simulink model "sampleModel1763"  (R2023a)
settings: Solver=VariableStepAuto  StartTime=0.0  StopTime=10.0  RelTol=1e-3
libraries: hdlsllib x4, simulink x1
settings Model: Creator=user1  LastModifiedBy=user1

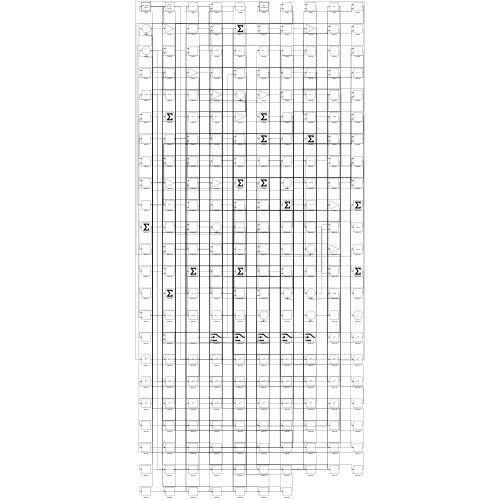
[thumbnail: Simulink's stored preview of the top-level diagram]
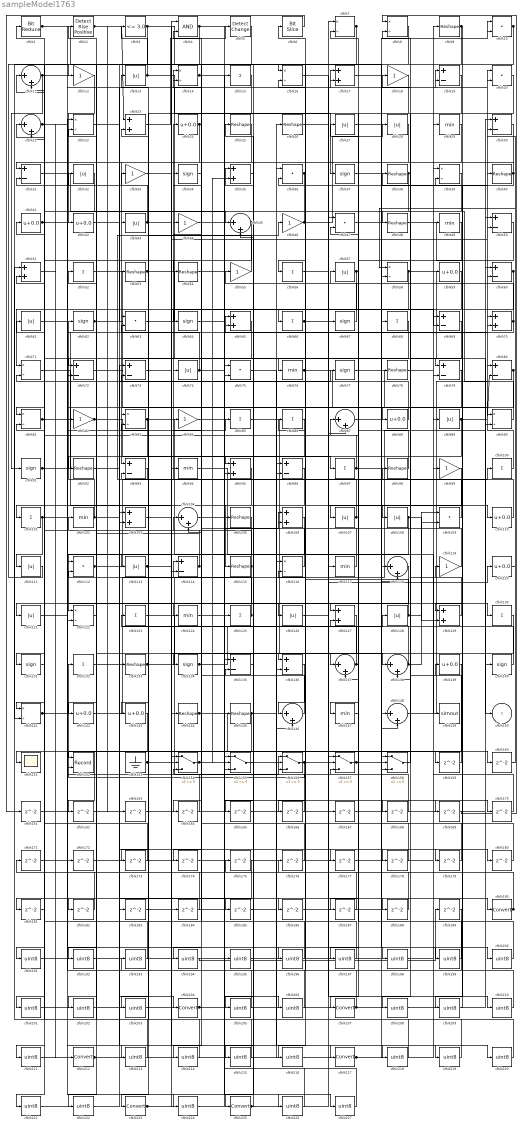
== system sampleModel1763 ==
  cfblk1 : hdlsllib/Logic and Bit Operations/Bit Reduce  mode=AND
  cfblk{10,20,36,47,63,75,109,112} (8 alike) : DotProduct  OutDataTypeStr=Inherit: Inherit via internal rule
  cfblk{15,52,56,66,68,85..86,97,100..101,123,125,130,132} (14 alike) : Sum  Inputs=+
  cfblk{29,49,76,94,102,117,124,147} (8 alike) : MinMax
  cfblk{17,23,35,51,65,70,95,103,106,127,129,136} (12 alike) : Sum
  cfblk{11,21,45,87,104,118,137..138,146,148} (10 alike) : Sum  Inputs=|++
  cfblk{9,25..26,38,40,48,53..54,78,92,98,105,115,133,144..145} (16 alike) : Reshape
  cfblk{13,27..28,32,43,57,61,74,89,107..108,111,113,121,126,128} (16 alike) : Abs  SaturateOnIntegerOverflow=off
  cfblk{24,41..42,59,88,110,120,139,142..143} (10 alike) : Bias  Bias=0.0  SaturateOnIntegerOverflow=off
  cfblk{19,30..31,50,60,69,72..73,79..80,93,96,114,135} (14 alike) : Sum  Inputs=+-
  cfblk{7..8,14,16,22,39,58,71,81,83,90,116,122,141} (14 alike) : Product  Inputs=*/  RndMeth=Zero  SaturateOnIntegerOverflow=on
  cfblk{12,18,33,44,46,55,82,84,99,119} (10 alike) : Gain
  cfblk{34,37,62,64,67,77,91,131,134,140} (10 alike) : Signum
  cfblk149 : ToWorkspace  VariableName=simout  SaveFormat=Timeseries  SampleTime=-1
  cfblk151 : Scope
  cfblk152 : Record  FileSettingsInternal="{\"entries\":[{\"content\":{\"excelSettings\":{\"content\":{},\"type\":\"Streamout.ExcelSettings\"}},\"type\":\"Streamout.FileSettingStorage\",\"uuid\":\"\"}],\"packageUris\":[\"http:\\/\\/schema.mathworks.com\\/mf0\\/streamout_blocks\\/R2020a\"],\"version\":\"1.0\"}"  Layout=[1 1]  SignalsInternal="{\"entries\":[{\"content\":{\"signals\":[{\"content\":{\"blockPath\":[],\"dimensions\":[1],\"domain\":\"\",\"lineColor\":\"#a2142f\",\"plots\":[1],\"port\":1,\"signalID\":3829,\"signalName\":\"XY Graph:1\"},\"type\":\"RecordBlkView.Signal\",\"uuid\":\"\"},{\"content\":{\"blockPath\":[],\"dimensions\":[1],\"domain\":\"\",\"lineColor\":\"#139fff\",\"plots\":[1],\"port\":2,\"signalID\":3832,\"signalName\":\"XY Graph:2\"},\"type\":\"RecordBlkView.Signal\",\"uuid\":\"\"}]},\"type\":\"RecordBlkView.InputSignals\",\"uuid\":\"\"}],\"packageUris\":[\"http:\\/\\/schema.mathworks.com\\/mf0\\/streamout_blocks\\/R2020a\"],\"version\":\"1.0\"}"  VisualizationBindings="{\"xyplotplugin\":{\"info\":[{\"series\":[{\"bindingParametersList\":[{\"parameter\":\"X-Axis\",\"signalID\":3829,\"signalName\":\"XY Graph:1\"},{\"parameter\":\"Y-Axis\",\"signalID\":3832,\"signalName\":\"XY Graph:2\"}],\"seriesID\":32770}],\"subplotID\":1}]}}"  CompatibilityTag=XY  st=-1
  cfblk153 : Ground
  cfblk{154..158} (5 alike) : Switch  SaturateOnIntegerOverflow=off  InputSameDT=off
  cfblk{159..189} (31 alike) : Delay  SampleTime=1
  cfblk{190,204,207,212,217,223,225} (7 alike) : DataTypeConversion  SaturateOnIntegerOverflow=off  RndMeth=Floor
  cfblk{191..203,205..206,208..211,213..216,218..222,224,226..227} (31 alike) : DataTypeConversion  OutDataTypeStr=uint8  SaturateOnIntegerOverflow=off  RndMeth=Floor
  cfblk2 : hdlsllib/Logic and Bit Operations/Detect Rise Positive  vinit=0  OutDataTypeStr=boolean
  cfblk3 : hdlsllib/Logic and Bit Operations/Compare To Constant  relop=<=  const=3.0  OutDataTypeStr=boolean
  cfblk4 : Logic  AllPortsSameDT=off  OutDataTypeStr=boolean
  cfblk5 : simulink/Logic and Bit Operations/Detect Change  vinit=0  OutDataTypeStr=boolean
      settings: LibrarySourceBlock=|
      | hdlsllib/Logic and Bit
      | Operations/Detect
      | Change
  cfblk6 : hdlsllib/Logic and Bit Operations/Bit Slice  lidx=7  ridx=0
  cfblk150 : Outport  VectorParamsAs1DForOutWhenUnconnected=off
  wires:
  cfblk59/1 -> cfblk93/1
  cfblk142/1 -> cfblk114/1
  cfblk140/1 -> cfblk102/1
  cfblk93/1 -> cfblk46/1
  cfblk48/1 -> cfblk107/1
  cfblk102/1 -> cfblk62/1, cfblk177/1
  cfblk90/1 -> cfblk48/1
  cfblk53/1 -> cfblk79/1, cfblk66/1
  cfblk12/1 -> cfblk42/1
  cfblk63/1 -> cfblk17/1
  cfblk60/1 -> cfblk71/1, cfblk129/1
  cfblk85/1 -> cfblk137/1
  cfblk136/1 -> cfblk146/1
  cfblk120/1 -> cfblk58/1
  cfblk100/1 -> cfblk20/1
  cfblk123/1 -> cfblk156/1
  cfblk30/1 -> cfblk83/1
  cfblk125/1 -> cfblk14/1, cfblk32/1
  cfblk134/1 -> cfblk7/1, cfblk169/1
  cfblk109/1 -> cfblk24/1
  cfblk146/1 -> cfblk44/1
  cfblk23/1 -> cfblk5/1
  cfblk67/1 -> cfblk57/1
  cfblk10/1 -> cfblk142/1, cfblk159/1
  cfblk148/1 -> cfblk80/1
  cfblk74/1 -> cfblk17/2, cfblk63/2, cfblk227/1
  cfblk31/1 -> cfblk125/1
  cfblk110/1 -> cfblk86/1
  cfblk22/1 -> cfblk204/1
  cfblk21/1 -> cfblk172/1, cfblk198/1
  cfblk46/1 -> cfblk28/1, cfblk43/1
  cfblk156/1 -> cfblk132/1, cfblk120/1
  cfblk116/1 -> cfblk34/1
  cfblk62/1 -> cfblk88/1, cfblk20/2
  cfblk133/1 -> cfblk30/1, cfblk23/2
  cfblk115/1 -> cfblk104/1, cfblk203/1
  cfblk73/1 -> cfblk217/1
  cfblk89/1 -> cfblk80/2, cfblk95/2
  cfblk105/1 -> cfblk122/1
  cfblk50/1 -> cfblk147/1
  cfblk28/1 -> cfblk64/1
  cfblk83/1 -> cfblk155/1, cfblk50/2, cfblk192/1
  cfblk129/1 -> cfblk38/1
  cfblk101/1 -> cfblk111/1, cfblk85/1
  cfblk71/1 -> cfblk144/1
  cfblk56/1 -> cfblk117/1
  cfblk58/1 -> cfblk150/1, cfblk222/1
  cfblk112/1 -> cfblk59/1, cfblk77/1
  cfblk14/1 -> cfblk134/1, cfblk168/1
  cfblk69/1 -> cfblk108/1
  cfblk138/1 -> cfblk123/1, cfblk109/2
  cfblk108/1 -> cfblk129/2, cfblk164/1
  cfblk57/1 -> cfblk113/1, cfblk137/2
  cfblk81/1 -> cfblk29/1, cfblk9/1
  cfblk141/1 -> cfblk213/1, cfblk224/1
  cfblk155/1 -> cfblk96/2
  cfblk32/1 -> cfblk81/1
  cfblk11/1 -> cfblk91/1, cfblk14/2
  cfblk95/1 -> cfblk121/1
  cfblk158/1 -> cfblk8/2
  cfblk77/1 -> cfblk90/1
  cfblk119/1 -> cfblk35/1
  cfblk66/1 -> cfblk126/1, cfblk180/1
  cfblk24/1 -> cfblk124/1, cfblk141/1
  cfblk145/1 -> cfblk152/1, cfblk194/1, cfblk219/1
  cfblk154/1 -> cfblk98/1, cfblk35/2
  cfblk157/1 -> cfblk19/1, cfblk70/1
  cfblk2/1 -> cfblk23/1, cfblk163/1
  cfblk135/1 -> cfblk225/1
  cfblk137/1 -> cfblk65/1, cfblk7/2
  cfblk144/1 -> cfblk158/2, cfblk128/1, cfblk106/2
  cfblk86/1 -> cfblk152/2
  cfblk43/1 -> cfblk45/1, cfblk31/2
  cfblk36/1 -> cfblk56/1, cfblk173/1
  cfblk70/1 -> cfblk65/2, cfblk16/2
  cfblk13/1 -> cfblk37/1, cfblk3/1
  cfblk79/1 -> cfblk122/2
  cfblk128/1 -> cfblk18/1, cfblk106/1, cfblk109/1
  cfblk44/1 -> cfblk97/1
  cfblk16/1 -> cfblk110/1
  cfblk82/1 -> cfblk145/1, cfblk130/1
  cfblk45/1 -> cfblk151/1, cfblk63/1, cfblk143/1
  cfblk96/1 -> cfblk115/1
  cfblk39/1 -> cfblk207/1
  cfblk94/1 -> cfblk149/1
  cfblk147/1 -> cfblk27/1
  cfblk3/1 -> cfblk148/2, cfblk141/2, cfblk185/1
  cfblk88/1 -> cfblk21/1
  cfblk132/1 -> cfblk94/1
  cfblk41/1 -> cfblk114/2, cfblk82/1
  cfblk153/1 -> cfblk83/2, cfblk127/2
  cfblk4/1 -> cfblk136/1, cfblk92/1
  cfblk131/1 -> cfblk21/2
  cfblk75/1 -> cfblk190/1
  cfblk52/1 -> cfblk76/1
  cfblk37/1 -> cfblk118/1
  cfblk33/1 -> cfblk69/2
  cfblk47/1 -> cfblk40/1
  cfblk15/1 -> cfblk223/1
  cfblk98/1 -> cfblk55/1
  cfblk19/1 -> cfblk53/1
  cfblk51/1 -> cfblk212/1
  cfblk113/1 -> cfblk138/1, cfblk100/1
  cfblk34/1 -> cfblk4/2
  cfblk107/1 -> cfblk33/1, cfblk74/1
  cfblk1/1 -> cfblk16/1, cfblk133/1, cfblk196/1, cfblk226/1
  cfblk7/1 -> cfblk54/1, cfblk72/1
  cfblk111/1 -> cfblk12/1
  cfblk121/1 -> cfblk127/1
  cfblk114/1 -> cfblk61/1, cfblk2/1
  cfblk80/1 -> cfblk104/2, cfblk166/1
  cfblk91/1 -> cfblk60/2, cfblk70/2
  cfblk9/1 -> cfblk95/1, cfblk209/1
  cfblk40/1 -> cfblk31/1, cfblk36/2
  cfblk65/1 -> cfblk131/1
  cfblk76/1 -> cfblk140/1, cfblk178/1
  cfblk64/1 -> cfblk90/2
  cfblk78/1 -> cfblk10/1
  cfblk122/1 -> cfblk52/1
  cfblk38/1 -> cfblk138/2, cfblk101/1
  cfblk117/1 -> cfblk25/1
  cfblk97/1 -> cfblk10/2, cfblk11/2
  cfblk55/1 -> cfblk13/1
  cfblk72/1 -> cfblk157/2
  cfblk17/1 -> cfblk19/2
  cfblk159/1 -> cfblk96/1
  cfblk61/1 -> cfblk160/1
  cfblk160/1 -> cfblk30/2
  cfblk6/1 -> cfblk161/1
  cfblk161/1 -> cfblk4/1
  cfblk139/1 -> cfblk162/1
  cfblk162/1 -> cfblk155/2
  cfblk163/1 -> cfblk136/2
  cfblk164/1 -> cfblk112/1
  cfblk35/1 -> cfblk165/1
  cfblk165/1 -> cfblk58/2
  cfblk166/1 -> cfblk156/2
  cfblk167/1 -> cfblk60/1
  cfblk168/1 -> cfblk93/2
  cfblk169/1 -> cfblk8/1
  cfblk54/1 -> cfblk170/1
  cfblk170/1 -> cfblk69/1
  cfblk171/1 -> cfblk47/1
  cfblk172/1 -> cfblk72/2
  cfblk173/1 -> cfblk11/1
  cfblk25/1 -> cfblk174/1
  cfblk174/1 -> cfblk79/2
  cfblk176/1 -> cfblk154/3
  cfblk177/1 -> cfblk158/3
  cfblk178/1 -> cfblk156/3
  cfblk126/1 -> cfblk179/1
  cfblk179/1 -> cfblk157/1
  cfblk180/1 -> cfblk157/3
  cfblk29/1 -> cfblk181/1
  cfblk181/1 -> cfblk71/2
  cfblk127/1 -> cfblk182/1
  cfblk182/1 -> cfblk81/2
  cfblk183/1 -> cfblk155/3
  cfblk184/1 -> cfblk154/1
  cfblk185/1 -> cfblk146/2
  cfblk124/1 -> cfblk186/1
  cfblk186/1 -> cfblk158/1
  cfblk18/1 -> cfblk187/1
  cfblk187/1 -> cfblk1/1
  cfblk92/1 -> cfblk188/1
  cfblk188/1 -> cfblk116/2
  cfblk190/1 -> cfblk139/1, cfblk6/1
  cfblk5/1 -> cfblk191/1
  cfblk191/1 -> cfblk75/1
  cfblk192/1 -> cfblk75/2
  cfblk189/1 -> cfblk193/1
  cfblk193/1 -> cfblk41/1
  cfblk194/1 -> cfblk189/1
  cfblk84/1 -> cfblk195/1
  cfblk195/1 -> cfblk148/1
  cfblk196/1 -> cfblk84/1
  cfblk49/1 -> cfblk197/1
  cfblk197/1 -> cfblk171/1
  cfblk198/1 -> cfblk49/1
  cfblk87/1 -> cfblk199/1
  cfblk199/1 -> cfblk47/2
  cfblk27/1 -> cfblk200/1
  cfblk200/1 -> cfblk87/1
  cfblk143/1 -> cfblk201/1
  cfblk201/1 -> cfblk87/2
  cfblk68/1 -> cfblk202/1
  cfblk202/1 -> cfblk116/1
  cfblk203/1 -> cfblk68/1
  cfblk204/1 -> cfblk167/1, cfblk50/1
  cfblk130/1 -> cfblk205/1
  cfblk205/1 -> cfblk22/1
  cfblk104/1 -> cfblk206/1
  cfblk206/1 -> cfblk22/2
  cfblk207/1 -> cfblk176/1, cfblk175/1, cfblk36/1
  cfblk20/1 -> cfblk208/1
  cfblk208/1 -> cfblk39/1
  cfblk209/1 -> cfblk39/2
  cfblk26/1 -> cfblk210/1
  cfblk210/1 -> cfblk119/1
  cfblk118/1 -> cfblk211/1
  cfblk211/1 -> cfblk26/1
  cfblk212/1 -> cfblk183/1, cfblk118/2
  cfblk213/1 -> cfblk51/1
  cfblk106/1 -> cfblk214/1
  cfblk214/1 -> cfblk51/2
  cfblk99/1 -> cfblk215/1
  cfblk215/1 -> cfblk112/2
  cfblk8/1 -> cfblk216/1
  cfblk216/1 -> cfblk99/1
  cfblk217/1 -> cfblk78/1, cfblk89/1
  cfblk42/1 -> cfblk218/1
  cfblk218/1 -> cfblk73/1
  cfblk219/1 -> cfblk73/2
  cfblk103/1 -> cfblk220/1
  cfblk220/1 -> cfblk154/2
  cfblk175/1 -> cfblk221/1
  cfblk221/1 -> cfblk103/1
  cfblk222/1 -> cfblk103/2
  cfblk223/1 -> cfblk184/1, cfblk105/1
  cfblk224/1 -> cfblk15/1
  cfblk225/1 -> cfblk45/2, cfblk67/1
  cfblk226/1 -> cfblk135/1
  cfblk227/1 -> cfblk135/2
